simulink model "atrias_boom_nmStand_fullCtrl"  (R2015a)
settings: Solver=ode23t  StartTime=0.0  StopTime=t_end  FixedStep=0.001  MaxStep=1e-3  RelTol=1e-3
InitFcn:
  | addpath('../common/')
  | colors
StartFcn:
  | tic
StopFcn:
  | %stopscript
values from neighbouring files (symbols this model uses):
  A1_notch_f1 = -2*cos(fnotch_f1*sample_time)    [set_control_params.m]
  A2_notch_f1 = 1    [set_control_params.m]
  A_lpf_dtau = 1 + B1_lpf_dtau + B2_lpf_dtau    [set_control_params.m]
  ankle_stiffness = 1/2*pi    (= 1.57079632679)    [mechanical_params.m]
  B1_lpf_dtau = -2*exp(-lpf_damping*fcut_dtau*sample_time)*cos(fcut_dtau*sample_time*sqrt(1-lpf_damping^2))    [set_control_params.m]
  B1_notch_f1 = -2*exp(-notch_damping*fnotch_f1*sample_time)*cos(fnotch_f1*sample_time*sqrt(1-notch_damping^2))    [set_control_params.m]
  B2_lpf_dtau = exp(-2*lpf_damping*fcut_dtau*sample_time)    [set_control_params.m]
  B2_notch_f1 = exp(-2*notch_damping*fnotch_f1*sample_time)    [set_control_params.m]
  b_hmotor = 0    [mechanical_params.m]
  b_leg_spring = 0.075*sqrt(k_leg_spring*0.5*.25^2)    [mechanical_params.m]
  b_rotor = 0*60/(2*pi)*9.725e-5    (= 0)    [mechanical_params.m]
  boom_mount_to_center_diagonal = boom_mount_to_center / cos(pitch_mount_angle)    [mechanical_params.m]    (also in set_control_params.m)
  breakaway_friction = [25 25 25 25]    [mechanical_params.m]
  contactThr = 0.35    [set_control_params.m]
  coulomb_friction = [20 20 20 20]    [mechanical_params.m]
  d_com = (d_hip_com_to_torso_com*m_torso)/(m_torso + num_legs*m_hshaft)    [mechanical_params.m]
  delta_phi_max = 160*pi/180    (= 2.79252680319)    [mechanical_params.m]    (also in set_control_params.m)
  delta_phi_max_buffer = 20*pi/180    (= 0.349065850399)    [set_control_params.m]
  delta_phi_max_dropoff = 2*pi/180    (= 0.0349065850399)    [set_control_params.m]
  delta_phi_min = 25.5*pi/180    (= 0.445058959259)    [mechanical_params.m]    (also in set_control_params.m)
  friction_linear_zone = [0.5 0.5 0.5 0.5].*pi/180    [mechanical_params.m]
  g = 9.803    [mechanical_params.m]    (also in set_control_params.m = 9.81)
  gain_nodes_sea_torque = [0,65,350,700]    [set_control_params.m]
  HIP_MTR_MAX_CONT_TORQUE = HIP_MTR_MAX_CONT_CURRENT*HIP_MOTOR_CONSTANT*HIP_MTR_GEAR_RATIO    (= 86.0016)    [set_control_params.m]
  HIP_MTR_MAX_TORQUE = max_current_hip*Kt_hip*N_h    (= 629.28)    [mechanical_params.m]
  initial_boom_pitch = 0    [mechanical_params.m]
  initial_boom_roll = asin((initial_com_height + boom_mount_to_com + boom_mount_to_center*tan(pitch_mount_angle) - (base_12(2) + yshaft_12(2))) / (l_boom + boom_mount_to_center_diagonal))    [mechanical_params.m]
  initial_boom_yaw = 0    [mechanical_params.m]
  initial_hip_roll = 0*pi/180    (= 0)    [mechanical_params.m]
  initial_winch_angle = -12 * pi/180    (= -0.209439510239)    [mechanical_params.m]
  k_gn = m_total*g/0.01    (= 57041.421916)    [mechanical_params.m]
  k_gt = m_total*g/0.1    (= 5704.1421916)    [mechanical_params.m]
  k_leg_spring = 4118.3    [mechanical_params.m]    (also in set_control_params.m)
  K_notch_f1 = (1+B1_notch_f1+B2_notch_f1)/(1+A1_notch_f1+A2_notch_f1)    [set_control_params.m]
  k_phi = 5000    [mechanical_params.m]
  k_sea = [4118.3 4118.3 4118.3 4118.3]    [set_control_params.m]
  Kb_leg = 0.121    [mechanical_params.m]
  kd_boom_roll_Ctrl = 0    [main_1_nmStand.m]    (also in main_2_nmStand_moveBoom.m)
  kd_lateral = 2*sqrt(kp_lateral*0.8)    [set_control_params.m]
  kd_shin_max = kd_pd_avoid_limits    (= 1000)    [set_control_params.m]
  kd_shin_min = kd_pd_avoid_limits    (= 1000)    [set_control_params.m]
  kd_splay_max = kd_pd_avoid_limits    (= 1000)    [set_control_params.m]
  kd_splay_min = kd_pd_avoid_limits    (= 1000)    [set_control_params.m]
  kd_thigh_max = kd_pd_avoid_limits    (= 1000)    [set_control_params.m]
  kd_thigh_min = kd_pd_avoid_limits    (= 1000)    [set_control_params.m]
  kd_winch = td_winch*kp_winch    (= 989.239577798)    [mechanical_params.m]
  kp_boom_roll_Ctrl = 0    [main_1_nmStand.m]    (also in main_2_nmStand_moveBoom.m)
  kp_lateral = 1000    [set_control_params.m]
  kp_sea_torque = [0.3, 0.3, 6.0, 6.0]    [set_control_params.m]
  kp_shin_max = kp_pd_avoid_limits    (= 5000)    [set_control_params.m]
  kp_shin_min = kp_pd_avoid_limits    (= 5000)    [set_control_params.m]
  kp_splay_max = kp_pd_avoid_limits    (= 5000)    [set_control_params.m]
  kp_splay_min = kp_pd_avoid_limits/10    (= 500)    [set_control_params.m]
  kp_thigh_max = kp_pd_avoid_limits    (= 5000)    [set_control_params.m]
  kp_thigh_min = kp_pd_avoid_limits    (= 5000)    [set_control_params.m]
  kp_winch = winch_gravity_comp/(3*pi/180)    (= 19784.791556)    [mechanical_params.m]
  Kt_leg = 0.121    [mechanical_params.m]
  l_boom = 1.8161    [mechanical_params.m]    (also in set_control_params.m)
  L_leg = 0.102e-3    (= 0.000102)    [mechanical_params.m]
  l_seg = 0.5    [mechanical_params.m]    (also in set_control_params.m)
  l_v = l_seg*cos(min_splay_angle/2)    [set_control_params.m]
  lateral_offset = 0.2    [set_control_params.m]
  lateral_target_angle_right = -6*pi/180    (= -0.10471975512)    [set_control_params.m]
  lateral_transition_force = 150    [set_control_params.m]
  LEG_MTR_MAX_TORQUE = max_current_leg * Kt_leg * N    (= 1210)    [mechanical_params.m]
  loaded_unloaded_torque_threshold = 65*ones(1,4)    [set_control_params.m]
  lowerleg_12 = 0.40    (= 0.4)    [mechanical_params.m]
  m_boom = 4.49    [mechanical_params.m]
  m_fblink = 0.46    [mechanical_params.m]    (also in set_control_params.m)
  m_foot = 0.0857    [mechanical_params.m]
  m_hshaft = 18    [mechanical_params.m]    (also in set_control_params.m = 20)
  m_leg = m_thigh + m_lowerleg + m_shin + m_fblink    (= 2.3438)    [mechanical_params.m]
  m_leg_motor = 18    [set_control_params.m]
  m_lowerleg = 0.4438    [mechanical_params.m]    (also in set_control_params.m)
  m_output_gear = 1e-5    (= 1e-05)    [mechanical_params.m]    (also in set_control_params.m)
  m_rotor = 1e-5    (= 1e-05)    [mechanical_params.m]    (also in set_control_params.m)
  m_shin = 0.75    [mechanical_params.m]    (also in set_control_params.m)
  m_thigh = 0.69    [mechanical_params.m]    (also in set_control_params.m)
  m_torso = 17.5    [mechanical_params.m]    (also in set_control_params.m = 17.9)
  m_total = num_legs*(m_hshaft + m_thigh + m_lowerleg + m_shin + m_fblink + 2*m_gearing) + m_torso    (= 58.18772)    [mechanical_params.m]    (also in set_control_params.m = 62.58772)
  m_virtual_gear = 1e-5    (= 1e-05)    [mechanical_params.m]    (also in set_control_params.m)
  m_yshaft = 12.89    [mechanical_params.m]
  max_current_leg = 200    [mechanical_params.m]
  max_sagittal_loaded_torque = 833    [set_control_params.m]
  max_sagittal_unloaded_torque = 267    [set_control_params.m]
  max_torque_lateral = min(MTR_HIP_MAX_CURRENT, HIP_CURRENT_LIMIT)*HIP_MOTOR_CONSTANT*HIP_MTR_GEAR_RATIO    [set_control_params.m]
  max_voltage_leg = 50    [mechanical_params.m]
  maximum_lateral_angle = 18*pi/180    (= 0.314159265359)    [set_control_params.m]
  min_splay_angle = 45*pi/180    (= 0.785398163397)    [set_control_params.m]
  min_splay_buffer = 1*pi/180    (= 0.0174532925199)    [set_control_params.m]
  min_splay_dropoff = 5*pi/180    (= 0.0872664625997)    [set_control_params.m]
  minimum_lateral_angle = -9.5*pi/180    (= -0.165806278939)    [set_control_params.m]
  mu_hmotor = 0.90    (= 0.9)    [mechanical_params.m]
  mu_motor = 0.85    [mechanical_params.m]
  mu_slide = 0.8    [mechanical_params.m]
  mu_stick = 0.9    [mechanical_params.m]
  N = 50    [mechanical_params.m]
  N_h = r_hip_shaft / r_hip_gearhead    (= 57)    [mechanical_params.m]
  phi_max_collision = -5*pi/180    (= -0.0872664625997)    [mechanical_params.m]
  phi_roll_max = pi + 16*pi/180    (= 3.42084533391)    [mechanical_params.m]
  phi_roll_min = pi - 9*pi/180    (= 2.98451302091)    [mechanical_params.m]
  phi_shin_max = 3*pi/2 + 17.5*pi/180    (= 5.01782159948)    [mechanical_params.m]    (also in set_control_params.m)
  phi_shin_max_buffer = 20*pi/180    (= 0.349065850399)    [set_control_params.m]
  phi_shin_max_dropoff = 2*pi/180    (= 0.0349065850399)    [set_control_params.m]
  phi_shin_min = pi - 45*pi/180    (= 2.35619449019)    [mechanical_params.m]    (also in set_control_params.m)
  phi_shin_min_buffer = 20*pi/180    (= 0.349065850399)    [set_control_params.m]
  phi_shin_min_dropoff = 2*pi/180    (= 0.0349065850399)    [set_control_params.m]
  phi_thigh_max = pi + 45*pi/180    (= 3.92699081699)    [mechanical_params.m]    (also in set_control_params.m)
  phi_thigh_max_buffer = 20*pi/180    (= 0.349065850399)    [set_control_params.m]
  phi_thigh_max_dropoff = 2*pi/180    (= 0.0349065850399)    [set_control_params.m]
  phi_thigh_min = pi/2 - 17.5*pi/180    (= 1.2653637077)    [mechanical_params.m]    (also in set_control_params.m)
  phi_thigh_min_buffer = 20*pi/180    (= 0.349065850399)    [set_control_params.m]
  phi_thigh_min_dropoff = 2*pi/180    (= 0.0349065850399)    [set_control_params.m]
  r_hip_gearhead = 0.009525    [mechanical_params.m]
  r_hip_shaft = 0.542925    [mechanical_params.m]
  R_leg = 0.052    [mechanical_params.m]
  r_rotor = 0.001    [mechanical_params.m]
  r_virtual_gear = N*r_rotor    (= 0.05)    [mechanical_params.m]
  releaseThr = 0.2    [set_control_params.m]
  sample_time = 0.001    [set_control_params.m]
  ... (+19 more)
undefined symbols (not defined in the file or in its folder): A_lpf_velocity, B1_lpf_velocity, B2_lpf_velocity, base_color_d, boom_color_d, c, c_jointstop, CtrlPar_theta0, eref, fblink_color_d, floor_color_d, FmaxBFSH, FmaxGLU, FmaxHAM, FmaxHFL, FmaxRF, FmaxVAS, foot_color_d, FPCtrlPar, hshaft_color_d, j_motor, K, lateral_motor_efficiency, LLCtrlPar, loptBFSH, loptGLU, loptHAM, loptHFL, loptRF, loptVAS, lowerleg_color_d, lslackBFSH, lslackGLU, lslackHAM, lslackHFL, lslackRF, lslackVAS, MidDelay_discrete, Newton, output_sample_time, phi12_max, phi12_min, phi23_max, phi23_min, phimaxRFk, phimaxVAS, phirefBFSH, phirefGLU, phirefHAMh, phirefHAMk, phirefHFL, phirefRFh, phirefRFk, phirefVAS, phiScaleRFk, phiScaleVAS, rad ... (+40)
libraries: sm_lib x210, nesl_utility x140, simulink x58, simulink_extras x26, fl_lib x16, mblibv1 x2, commnoisgen2 x1
(part 18 of 19)

== system atrias_boom_nmStand_fullCtrl/Control/Behavior Control/Virtual Neuromuscular Control/Neural Control Layer/R Swing Phase (sagittal)/kneeii_damp and hold &kneeiii_leg stop &kneeiv_stance preparation ==
  note: Knee Phase i
  CtrlPar : Inport
  a_tgt : Inport  Port=2
  a : Inport  Port=3
  da : Inport  Port=4
  phiH : Inport  Port=5
  phiK : Inport  Port=6
  dphiK : Inport  Port=7
  Enable : EnablePort  StatesWhenEnabling=reset
  Constant1 : Constant  Value=0  OutDataTypeStr=boolean
  Constant2 : Constant  Value=0  OutDataTypeStr=boolean
  Constant3 : Constant  Value=0  OutDataTypeStr=boolean
  Demux1 : Demux  Outputs=2
  Logical Operator : Logic  Operator=NOT  AllPortsSameDT=off  OutDataTypeStr=boolean
  Logical Operator1 : Logic  AllPortsSameDT=off  OutDataTypeStr=boolean
  Mux : Mux  Inputs=3
  Relational Operator : RelationalOperator  Operator=<=  OutDataTypeStr=boolean
  Relational Operator1 : RelationalOperator  Operator=<=  OutDataTypeStr=boolean
  Relational Operator2 : RelationalOperator  OutDataTypeStr=boolean
  S-R Flip-Flop : simulink_extras/Flip Flops/S-R Flip-Flop  initial_condition=0
  S-R Flip-Flop1 : simulink_extras/Flip Flops/S-R Flip-Flop  initial_condition=0
  S-R Flip-Flop2 : simulink_extras/Flip Flops/S-R Flip-Flop  initial_condition=0
  Sum2 : Sum  Inputs=++|  SaturateOnIntegerOverflow=on  InputSameDT=on  OutDataTypeStr=Inherit: Same as first input
  Terminator : Terminator
  Terminator1 : Terminator
  Terminator2 : Terminator
  kneeii_damp and hold : Subsystem  TreatAsAtomicUnit=on
  kneeiii_leg stop : Subsystem  TreatAsAtomicUnit=on
  kneeiv_stance preparation : Subsystem  TreatAsAtomicUnit=on
  parSwKii : Selector  InputPortWidth=Sw_i  Indices=parSwKii_i
  parSwKiii : Selector  InputPortWidth=Sw_i  Indices=parSwKiii_i
  parSwKiv : Selector  InputPortWidth=Sw_i  Indices=parSwKiv_i
  parSwPhii : Selector  InputPortWidth=Sw_i  Indices=parSwPh_i
  phase [M8 M9 M10] : Outport  OutputWhenDisabled=reset  InitialOutput=0
  SRF_Sw_kii : Outport  Port=2  OutputWhenDisabled=reset  InitialOutput=0
  SVAS_Sw_kii : Outport  Port=3  OutputWhenDisabled=reset  InitialOutput=0
  SBFSH_Sw_kii : Outport  Port=4  OutputWhenDisabled=reset  InitialOutput=0
  SHAM_Sw_kiii : Outport  Port=5  OutputWhenDisabled=reset  InitialOutput=0
  SBFSH_Sw_kiii : Outport  Port=6  OutputWhenDisabled=reset  InitialOutput=0
  SHFL_Sw_kiv : Outport  Port=7  OutputWhenDisabled=reset  InitialOutput=0
  SGLU_Sw_kiv : Outport  Port=8  OutputWhenDisabled=reset  InitialOutput=0
  SVAS_Sw_kiv : Outport  Port=9  OutputWhenDisabled=reset  InitialOutput=0
  wires:
  phiK/1 -> kneeiv_stance preparation/4(phiK)
  phiH/1 -> kneeiv_stance preparation/3(phiH)
  dphiK/1 -> kneeii_damp and hold/5(dphiK)
  da/1 -> Relational Operator2/1, kneeii_damp and hold/4(da)
  Sum2/1 -> Relational Operator1/2  "a_thr"
  a/1 -> Relational Operator/1, Relational Operator1/1, kneeiii_leg stop/3(a), kneeii_damp and hold/3("a ")
  Mux/1 -> phase [M8 M9 M10]/1
  Relational Operator2/1 -> Logical Operator1/2
  Logical Operator/1 -> Mux/1, kneeii_damp and hold/Enable
  a_tgt/1 -> kneeiv_stance preparation/2(a_tgt), kneeiii_leg stop/2(a_tgt), kneeii_damp and hold/2(a_tgt), Relational Operator/2, Sum2/1
  kneeiv_stance preparation/3(SVAS_Sw_kiv) -> SVAS_Sw_kiv/1
  kneeiv_stance preparation/2(SGLU_Sw_kiv) -> SGLU_Sw_kiv/1
  kneeiv_stance preparation/1(SHFL_Sw_kiv) -> SHFL_Sw_kiv/1
  kneeiii_leg stop/2(SBFSH_Sw_kiii) -> SBFSH_Sw_kiii/1
  kneeiii_leg stop/1(SHAM_Sw_kiii) -> SHAM_Sw_kiii/1
  kneeii_damp and hold/3(SBFSH_Sw_kii) -> SBFSH_Sw_kii/1
  kneeii_damp and hold/1(SRF_Sw_kii) -> SRF_Sw_kii/1
  parSwKiv/1 -> kneeiv_stance preparation/1(CtrlPar)
  parSwKiii/1 -> kneeiii_leg stop/1(CtrlPar)
  S-R Flip-Flop2/1 -> kneeiv_stance preparation/Enable, Mux/3
  S-R Flip-Flop1/1 -> Logical Operator1/1, kneeiii_leg stop/Enable, Mux/2
  parSwKii/1 -> kneeii_damp and hold/1(CtrlPar)
  S-R Flip-Flop/1 -> Logical Operator/1
  CtrlPar/1 -> parSwKiv/1, parSwKiii/1, parSwKii/1, parSwPhii/1
  Logical Operator1/1 -> S-R Flip-Flop2/1
  S-R Flip-Flop2/2 -> Terminator2/1
  Constant3/1 -> S-R Flip-Flop2/2
  Relational Operator1/1 -> S-R Flip-Flop1/1
  S-R Flip-Flop1/2 -> Terminator1/1
  Constant2/1 -> S-R Flip-Flop1/2
  Relational Operator/1 -> S-R Flip-Flop/1
  S-R Flip-Flop/2 -> Terminator/1
  Constant1/1 -> S-R Flip-Flop/2
  Demux1/1 -> Sum2/2  "Sw_a_del"
  parSwPhii/1 -> Demux1/1
  Demux1/2 -> Relational Operator2/2  "Sw_da_del"
  kneeii_damp and hold/2(SVAS_Sw_kii) -> SVAS_Sw_kii/1

== system atrias_boom_nmStand_fullCtrl/Control/Behavior Control/Virtual Neuromuscular Control/Torque Distribution/mech limit avoidance1/PD Joint Limit ==
  L Mechanical Limit Avoidance Torque : Subsystem
  L scale desired torque : Subsystem
  Mux1 : Mux
  Mux2 : Mux
  R Mechanical Limit Avoidance Torque : Subsystem
  R scale desired torque : Subsystem
  tau_pd_hip_knee [Nm]x4 : Outport
  des_trq_scale x4 : Outport  Port=2
  tag scope: L_scale_hip=global, L_scale_knee=global, Ltau_pd_hip=global, Ltau_pd_knee=global, R_scale_hip=global, R_scale_knee=global, Rtau_pd_hip=global, Rtau_pd_knee=global
  wires:
  L scale desired torque/2(scale_knee) -> [L_scale_knee]
  L scale desired torque/1(scale_hip) -> [L_scale_hip]
  [Lphi_shin] -> L scale desired torque/2(phi_shin [rad])
  [Lphi_thigh] -> L scale desired torque/1(phi_thigh [rad])
  R Mechanical Limit Avoidance Torque/1(tau_pd_hip [Nm]) -> [Rtau_pd_hip]
  L Mechanical Limit Avoidance Torque/2(tau_pd_knee [Nm]) -> [Ltau_pd_knee]
  L Mechanical Limit Avoidance Torque/1(tau_pd_hip [Nm]) -> [Ltau_pd_hip]
  R Mechanical Limit Avoidance Torque/2(tau_pd_knee [Nm]) -> [Rtau_pd_knee]
  Mux2/1 -> tau_pd_hip_knee [Nm]x4/1
  [Rtau_pd_hip] -> Mux2/1
  [Rtau_pd_knee] -> Mux2/2
  [Ltau_pd_hip] -> Mux2/3
  [Ltau_pd_knee] -> Mux2/4
  Mux1/1 -> des_trq_scale x4/1
  [R_scale_hip] -> Mux1/1
  [R_scale_knee] -> Mux1/2
  [L_scale_hip] -> Mux1/3
  [L_scale_knee] -> Mux1/4
  R scale desired torque/2(scale_knee) -> [R_scale_knee]
  R scale desired torque/1(scale_hip) -> [R_scale_hip]
  [Rphi_shin] -> R scale desired torque/2(phi_shin [rad])
  [Rphi_thigh] -> R scale desired torque/1(phi_thigh [rad])
  [Rdphi_shin] -> R Mechanical Limit Avoidance Torque/4(dphi_shin [rad/s])
  [Rdphi_thigh] -> R Mechanical Limit Avoidance Torque/3(dphi_thigh [rad/s])
  [Rphi_shin] -> R Mechanical Limit Avoidance Torque/2(phi_shin [rad])
  [Rphi_thigh] -> R Mechanical Limit Avoidance Torque/1(phi_thigh [rad])
  [Ldphi_shin] -> L Mechanical Limit Avoidance Torque/4(dphi_shin [rad/s])
  [Ldphi_thigh] -> L Mechanical Limit Avoidance Torque/3(dphi_thigh [rad/s])
  [Lphi_shin] -> L Mechanical Limit Avoidance Torque/2(phi_shin [rad])
  [Lphi_thigh] -> L Mechanical Limit Avoidance Torque/1(phi_thigh [rad])

== system atrias_boom_nmStand_fullCtrl/Control/Behavior Control/Virtual Neuromuscular Control/Torque Distribution/mech limit avoidance1/PD Joint Limit1 ==
  Demux : Demux
  Lechanical Limit Avoidance Torques : Subsystem
  Mux1 : Mux
  R Mechanical Limit Avoidance Torque : Subsystem
  R scale desired torque : Subsystem
  R scale desired torque1 : Subsystem
  to hip_knee : MATLAB Function  TreatAsAtomicUnit=on
  tau_pd_hip_knee [Nm]x4 : Outport
  des_trq_scale x4 : Outport  Port=2
  tag scope: L_scale_hip=global, L_scale_knee=global, Ltau_pd_back=global, Ltau_pd_front=global, Ltau_pd_hip=global, Ltau_pd_knee=global, R_scale_hip=global, R_scale_knee=global, Rtau_pd_back=global, Rtau_pd_front=global, Rtau_pd_hip=global, Rtau_pd_knee=global
  wires:
  [Lphi_thigh] -> Lechanical Limit Avoidance Torques/1(phi_thigh [rad])
  [Lphi_shin] -> Lechanical Limit Avoidance Torques/2(phi_shin [rad])
  [Ldphi_thigh] -> Lechanical Limit Avoidance Torques/3(dphi_thigh [rad/s])
  [Ldphi_shin] -> Lechanical Limit Avoidance Torques/4(dphi_shin [rad/s])
  Lechanical Limit Avoidance Torques/1(tau_pd_back [Nm]) -> [Ltau_pd_back]
  Lechanical Limit Avoidance Torques/2(tau_pd_front [Nm]) -> [Ltau_pd_front]
  [Rphi_thigh] -> R Mechanical Limit Avoidance Torque/1(phi_thigh [rad])
  [Rphi_shin] -> R Mechanical Limit Avoidance Torque/2(phi_shin [rad])
  [Rdphi_thigh] -> R Mechanical Limit Avoidance Torque/3(dphi_thigh [rad/s])
  [Rdphi_shin] -> R Mechanical Limit Avoidance Torque/4(dphi_shin [rad/s])
  R Mechanical Limit Avoidance Torque/1(tau_pd_back [Nm]) -> [Rtau_pd_back]
  R Mechanical Limit Avoidance Torque/2(tau_pd_front [Nm]) -> [Rtau_pd_front]
  [Rphi_thigh] -> R scale desired torque/1(phi_thigh [rad])
  [Rphi_shin] -> R scale desired torque/2(phi_shin [rad])
  R scale desired torque/1(scale_hip) -> [R_scale_hip]
  R scale desired torque/2(scale_knee) -> [R_scale_knee]
  [k_R] -> to hip_knee/5(kR)
  [k_L] -> to hip_knee/6(kL)
  [Ltau_pd_front] -> to hip_knee/4(Ltau_front)
  [Ltau_pd_back] -> to hip_knee/3(Ltau_back)
  [Rtau_pd_front] -> to hip_knee/2(Rtau_front)
  [Rtau_pd_back] -> to hip_knee/1(Rtau_back)
  to hip_knee/1(tau_pd_hip_knee) -> tau_pd_hip_knee [Nm]x4/1, Demux/1
  [k_R] -> R scale desired torque/3(k)
  [Lphi_thigh] -> R scale desired torque1/1(phi_thigh [rad])
  [Lphi_shin] -> R scale desired torque1/2(phi_shin [rad])
  R scale desired torque1/1(scale_hip) -> [L_scale_hip]
  R scale desired torque1/2(scale_knee) -> [L_scale_knee]
  [k_L] -> R scale desired torque1/3(k)
  [L_scale_knee] -> Mux1/4
  [L_scale_hip] -> Mux1/3
  [R_scale_knee] -> Mux1/2
  [R_scale_hip] -> Mux1/1
  Mux1/1 -> des_trq_scale x4/1
  Demux/1 -> [Rtau_pd_hip]
  Demux/2 -> [Rtau_pd_knee]
  Demux/3 -> [Ltau_pd_hip]
  Demux/4 -> [Ltau_pd_knee]

== system atrias_boom_nmStand_fullCtrl/Mechanical System Layer/Ground Contact Models/L Back Ground Contact/3D Contact/Kinetic Friction Model/Vector Norm ==
  vec : Inport
  Sqrt : Sqrt  OutputSignalType=real  AlgorithmType=Newton-Raphson  SaturateOnIntegerOverflow=on
  Squares : Math  Operator=square  OutputSignalType=real  SaturateOnIntegerOverflow=on
  Sum of Elements : Sum  Inputs=+
  norm : Outport
  wires:
  vec/1 -> Squares/1
  Sqrt/1 -> norm/1
  Sum of Elements/1 -> Sqrt/1
  Squares/1 -> Sum of Elements/1

== system atrias_boom_nmStand_fullCtrl/Mechanical System Layer/Ground Contact Models/L Back Ground Contact/3D Contact/Static Friction Model/Vector Norm ==
  vec : Inport
  Sqrt : Sqrt  OutputSignalType=real  AlgorithmType=Newton-Raphson  SaturateOnIntegerOverflow=on
  Squares : Math  Operator=square  OutputSignalType=real  SaturateOnIntegerOverflow=on
  Sum of Elements : Sum  Inputs=+
  norm : Outport
  wires:
  vec/1 -> Squares/1
  Sqrt/1 -> norm/1
  Sum of Elements/1 -> Sqrt/1
  Squares/1 -> Sum of Elements/1

== system atrias_boom_nmStand_fullCtrl/Mechanical System Layer/Ground Contact Models/L Front Ground Contact/3D Contact/Kinetic Friction Model/Vector Norm ==
  vec : Inport
  Sqrt : Sqrt  OutputSignalType=real  AlgorithmType=Newton-Raphson  SaturateOnIntegerOverflow=on
  Squares : Math  Operator=square  OutputSignalType=real  SaturateOnIntegerOverflow=on
  Sum of Elements : Sum  Inputs=+
  norm : Outport
  wires:
  vec/1 -> Squares/1
  Sqrt/1 -> norm/1
  Sum of Elements/1 -> Sqrt/1
  Squares/1 -> Sum of Elements/1

== system atrias_boom_nmStand_fullCtrl/Mechanical System Layer/Ground Contact Models/L Front Ground Contact/3D Contact/Static Friction Model/Vector Norm ==
  vec : Inport
  Sqrt : Sqrt  OutputSignalType=real  AlgorithmType=Newton-Raphson  SaturateOnIntegerOverflow=on
  Squares : Math  Operator=square  OutputSignalType=real  SaturateOnIntegerOverflow=on
  Sum of Elements : Sum  Inputs=+
  norm : Outport
  wires:
  vec/1 -> Squares/1
  Sqrt/1 -> norm/1
  Sum of Elements/1 -> Sqrt/1
  Squares/1 -> Sum of Elements/1

== system atrias_boom_nmStand_fullCtrl/Mechanical System Layer/Ground Contact Models/R Back Ground Contact/3D Contact/Kinetic Friction Model/Vector Norm ==
  vec : Inport
  Sqrt : Sqrt  OutputSignalType=real  AlgorithmType=Newton-Raphson  SaturateOnIntegerOverflow=on
  Squares : Math  Operator=square  OutputSignalType=real  SaturateOnIntegerOverflow=on
  Sum of Elements : Sum  Inputs=+
  norm : Outport
  wires:
  vec/1 -> Squares/1
  Sqrt/1 -> norm/1
  Sum of Elements/1 -> Sqrt/1
  Squares/1 -> Sum of Elements/1

== system atrias_boom_nmStand_fullCtrl/Mechanical System Layer/Ground Contact Models/R Back Ground Contact/3D Contact/Static Friction Model/Vector Norm ==
  vec : Inport
  Sqrt : Sqrt  OutputSignalType=real  AlgorithmType=Newton-Raphson  SaturateOnIntegerOverflow=on
  Squares : Math  Operator=square  OutputSignalType=real  SaturateOnIntegerOverflow=on
  Sum of Elements : Sum  Inputs=+
  norm : Outport
  wires:
  vec/1 -> Squares/1
  Sqrt/1 -> norm/1
  Sum of Elements/1 -> Sqrt/1
  Squares/1 -> Sum of Elements/1

== system atrias_boom_nmStand_fullCtrl/Mechanical System Layer/Ground Contact Models/R Front Ground Contact/3D Contact/Kinetic Friction Model/Vector Norm ==
  vec : Inport
  Sqrt : Sqrt  OutputSignalType=real  AlgorithmType=Newton-Raphson  SaturateOnIntegerOverflow=on
  Squares : Math  Operator=square  OutputSignalType=real  SaturateOnIntegerOverflow=on
  Sum of Elements : Sum  Inputs=+
  norm : Outport
  wires:
  vec/1 -> Squares/1
  Sqrt/1 -> norm/1
  Sum of Elements/1 -> Sqrt/1
  Squares/1 -> Sum of Elements/1

== system atrias_boom_nmStand_fullCtrl/Mechanical System Layer/Ground Contact Models/R Front Ground Contact/3D Contact/Static Friction Model/Vector Norm ==
  vec : Inport
  Sqrt : Sqrt  OutputSignalType=real  AlgorithmType=Newton-Raphson  SaturateOnIntegerOverflow=on
  Squares : Math  Operator=square  OutputSignalType=real  SaturateOnIntegerOverflow=on
  Sum of Elements : Sum  Inputs=+
  norm : Outport
  wires:
  vec/1 -> Squares/1
  Sqrt/1 -> norm/1
  Sum of Elements/1 -> Sqrt/1
  Squares/1 -> Sum of Elements/1

== system atrias_boom_nmStand_fullCtrl/Control/Behavior Control/Virtual Neuromuscular Control/Neural Control Layer/L Swing Phase (sagittal)/kneeii_damp and hold &kneeiii_leg stop &kneeiv_stance preparation/kneeii_damp and hold ==
  note: Knee Phase i
  CtrlPar : Inport
  a_tgt : Inport  Port=2
  "a " : Inport  Port=3
  da : Inport  Port=4
  dphiK : Inport  Port=5
  Enable : EnablePort  StatesWhenEnabling=reset
  Demux2 : Demux
  Divide1 : Product
  Divide2 : Product  Inputs=3
  Divide3 : Product
  Divide5 : Product
  Gain3 : Gain  Gain=-1
  Sum2 : Sum  Inputs=|+-  SaturateOnIntegerOverflow=on  InputSameDT=on  OutDataTypeStr=Inherit: Same as first input
  Sum4 : Sum  Inputs=+-|  SaturateOnIntegerOverflow=on  InputSameDT=on  OutDataTypeStr=Inherit: Same as first input
  Sum7 : Sum  Inputs=++|  SaturateOnIntegerOverflow=on  InputSameDT=on  OutDataTypeStr=Inherit: Same as first input
  negative half : Saturate  UpperLimit=0  LowerLimit=-inf  ZeroCross=off
  positive half{,1..3} (4 alike) : Saturate  UpperLimit=inf  LowerLimit=0  ZeroCross=off
  SRF_Sw_kii : Outport  OutputWhenDisabled=reset  InitialOutput=0
  SVAS_Sw_kii : Outport  Port=2  OutputWhenDisabled=reset  InitialOutput=0
  SBFSH_Sw_kii : Outport  Port=3  OutputWhenDisabled=reset  InitialOutput=0
  wires:
  Demux2/4 -> Divide1/2  "Sw_dphiKGain_BFSH"
  Demux2/1 -> Divide5/2  "Sw_dphiKGain_RF"
  da/1 -> Sum7/2
  dphiK/1 -> negative half/1, Sum7/1, positive half/1
  a_tgt/1 -> Sum2/1
  Divide2/1 -> SBFSH_Sw_kii/1
  Sum2/1 -> positive half2/1
  "a "/1 -> Sum2/2
  positive half2/1 -> Divide2/3
  Sum7/1 -> positive half1/1
  positive half1/1 -> Divide2/2
  Divide1/1 -> Divide2/1
  positive half/1 -> Divide1/1
  Divide5/1 -> SRF_Sw_kii/1, Sum4/1
  CtrlPar/1 -> Demux2/1
  negative half/1 -> Gain3/1
  Gain3/1 -> Divide5/1
  positive half3/1 -> Divide3/1
  Sum4/1 -> positive half3/1
  Demux2/2 -> Sum4/2  "Sw_SRF_thr"
  Demux2/3 -> Divide3/2  "Sw_SGainRF_VAS"
  Divide3/1 -> SVAS_Sw_kii/1

== system atrias_boom_nmStand_fullCtrl/Control/Behavior Control/Virtual Neuromuscular Control/Neural Control Layer/L Swing Phase (sagittal)/kneeii_damp and hold &kneeiii_leg stop &kneeiv_stance preparation/kneeiii_leg stop ==
  note: Knee Phase iii
  CtrlPar : Inport
  a_tgt : Inport  Port=2
  a : Inport  Port=3
  Enable : EnablePort  StatesWhenEnabling=reset
  Demux2 : Demux
  Divide1 : Product
  Divide5 : Product
  Sum1 : Sum  Inputs=+-|  SaturateOnIntegerOverflow=on  InputSameDT=on  OutDataTypeStr=Inherit: Same as first input
  Sum2 : Sum  Inputs=++|  SaturateOnIntegerOverflow=on  InputSameDT=on  OutDataTypeStr=Inherit: Same as first input
  Sum4 : Sum  Inputs=+-|  SaturateOnIntegerOverflow=on  InputSameDT=on  OutDataTypeStr=Inherit: Same as first input
  positive half1 : Saturate  UpperLimit=inf  LowerLimit=0  ZeroCross=off
  positive half2 : Saturate  UpperLimit=inf  LowerLimit=0  ZeroCross=off
  SHAM_Sw_kiii : Outport  OutputWhenDisabled=reset  InitialOutput=0
  SBFSH_Sw_kiii : Outport  Port=2  OutputWhenDisabled=reset  InitialOutput=0
  wires:
  Demux2/1 -> Sum2/2  "Sw_a_del"
  a/1 -> Sum1/2
  Divide1/1 -> SBFSH_Sw_kiii/1
  Demux2/4 -> Divide1/2  "Sw_SGainHAM_BFSH"
  positive half1/1 -> Divide1/1
  Demux2/3 -> Sum4/2  "SHAM_thr"
  Sum4/1 -> positive half1/1
  Divide5/1 -> SHAM_Sw_kiii/1, Sum4/1  "S_HAM"
  Demux2/2 -> Divide5/2  "Sw_alpGain_HAM"
  Sum2/1 -> Sum1/1  "a_thr"
  a_tgt/1 -> Sum2/1
  positive half2/1 -> Divide5/1  "del_alp"
  Sum1/1 -> positive half2/1  "del_alp"
  CtrlPar/1 -> Demux2/1

== system atrias_boom_nmStand_fullCtrl/Control/Behavior Control/Virtual Neuromuscular Control/Neural Control Layer/L Swing Phase (sagittal)/kneeii_damp and hold &kneeiii_leg stop &kneeiv_stance preparation/kneeiv_stance preparation ==
  note: Knee Phase iii
  CtrlPar : Inport
  a_tgt : Inport  Port=2
  phiH : Inport  Port=3
  phiK : Inport  Port=4
  Enable : EnablePort  StatesWhenEnabling=reset
  Constant5 : Constant  Value=pi/2
  Demux1 : Demux
  Divide3 : Product
  Divide5 : Product
  Divide6 : Product
  Sum1 : Sum  Inputs=-+|  SaturateOnIntegerOverflow=on  InputSameDT=on  OutDataTypeStr=Inherit: Same as first input
  Sum2 : Sum  Inputs=++|  SaturateOnIntegerOverflow=on  InputSameDT=on  OutDataTypeStr=Inherit: Same as first input
  Sum9 : Sum  Inputs=+-|  SaturateOnIntegerOverflow=on  InputSameDT=on  OutDataTypeStr=Inherit: Same as first input
  positive half2 : Saturate  UpperLimit=inf  LowerLimit=0  ZeroCross=off
  positive half3 : Saturate  UpperLimit=inf  LowerLimit=0  ZeroCross=off
  SHFL_Sw_kiv : Outport  OutputWhenDisabled=reset  InitialOutput=0
  SGLU_Sw_kiv : Outport  Port=2  OutputWhenDisabled=reset  InitialOutput=0
  SVAS_Sw_kiv : Outport  Port=3  OutputWhenDisabled=reset  InitialOutput=0
  wires:
  Demux1/4 -> Divide6/2
  Demux1/3 -> Sum9/1
  Demux1/2 -> Divide3/1
  Demux1/1 -> Divide5/2
  phiH/1 -> Sum1/2
  Divide6/1 -> SVAS_Sw_kiv/1
  positive half3/1 -> Divide6/1
  phiK/1 -> Sum9/2
  Sum9/1 -> positive half3/1
  Divide3/1 -> SGLU_Sw_kiv/1
  positive half2/1 -> Divide5/1, Divide3/2
  Divide5/1 -> SHFL_Sw_kiv/1
  Sum2/1 -> Sum1/1
  Constant5/1 -> Sum2/1
  a_tgt/1 -> Sum2/2
  Sum1/1 -> positive half2/1
  CtrlPar/1 -> Demux1/1

== system atrias_boom_nmStand_fullCtrl/Control/Behavior Control/Virtual Neuromuscular Control/Neural Control Layer/R Swing Phase (sagittal)/kneeii_damp and hold &kneeiii_leg stop &kneeiv_stance preparation/kneeii_damp and hold ==
  note: Knee Phase i
  CtrlPar : Inport
  a_tgt : Inport  Port=2
  "a " : Inport  Port=3
  da : Inport  Port=4
  dphiK : Inport  Port=5
  Enable : EnablePort  StatesWhenEnabling=reset
  Demux2 : Demux
  Divide1 : Product
  Divide2 : Product  Inputs=3
  Divide3 : Product
  Divide5 : Product
  Gain3 : Gain  Gain=-1
  Sum2 : Sum  Inputs=|+-  SaturateOnIntegerOverflow=on  InputSameDT=on  OutDataTypeStr=Inherit: Same as first input
  Sum4 : Sum  Inputs=+-|  SaturateOnIntegerOverflow=on  InputSameDT=on  OutDataTypeStr=Inherit: Same as first input
  Sum7 : Sum  Inputs=++|  SaturateOnIntegerOverflow=on  InputSameDT=on  OutDataTypeStr=Inherit: Same as first input
  negative half : Saturate  UpperLimit=0  LowerLimit=-inf  ZeroCross=off
  positive half{,1..3} (4 alike) : Saturate  UpperLimit=inf  LowerLimit=0  ZeroCross=off
  SRF_Sw_kii : Outport  OutputWhenDisabled=reset  InitialOutput=0
  SVAS_Sw_kii : Outport  Port=2  OutputWhenDisabled=reset  InitialOutput=0
  SBFSH_Sw_kii : Outport  Port=3  OutputWhenDisabled=reset  InitialOutput=0
  wires:
  Demux2/4 -> Divide1/2  "Sw_dphiKGain_BFSH"
  Demux2/1 -> Divide5/2  "Sw_dphiKGain_RF"
  da/1 -> Sum7/2
  dphiK/1 -> negative half/1, Sum7/1, positive half/1
  a_tgt/1 -> Sum2/1
  Divide2/1 -> SBFSH_Sw_kii/1
  Sum2/1 -> positive half2/1
  "a "/1 -> Sum2/2
  positive half2/1 -> Divide2/3
  Sum7/1 -> positive half1/1
  positive half1/1 -> Divide2/2
  Divide1/1 -> Divide2/1
  positive half/1 -> Divide1/1
  Divide5/1 -> SRF_Sw_kii/1, Sum4/1
  CtrlPar/1 -> Demux2/1
  negative half/1 -> Gain3/1
  Gain3/1 -> Divide5/1
  positive half3/1 -> Divide3/1
  Sum4/1 -> positive half3/1
  Demux2/2 -> Sum4/2  "Sw_SRF_thr"
  Demux2/3 -> Divide3/2  "Sw_SGainRF_VAS"
  Divide3/1 -> SVAS_Sw_kii/1

== system atrias_boom_nmStand_fullCtrl/Control/Behavior Control/Virtual Neuromuscular Control/Neural Control Layer/R Swing Phase (sagittal)/kneeii_damp and hold &kneeiii_leg stop &kneeiv_stance preparation/kneeiii_leg stop ==
  note: Knee Phase iii
  CtrlPar : Inport
  a_tgt : Inport  Port=2
  a : Inport  Port=3
  Enable : EnablePort  StatesWhenEnabling=reset
  Demux2 : Demux
  Divide1 : Product
  Divide5 : Product
  Sum1 : Sum  Inputs=+-|  SaturateOnIntegerOverflow=on  InputSameDT=on  OutDataTypeStr=Inherit: Same as first input
  Sum2 : Sum  Inputs=++|  SaturateOnIntegerOverflow=on  InputSameDT=on  OutDataTypeStr=Inherit: Same as first input
  Sum4 : Sum  Inputs=+-|  SaturateOnIntegerOverflow=on  InputSameDT=on  OutDataTypeStr=Inherit: Same as first input
  positive half1 : Saturate  UpperLimit=inf  LowerLimit=0  ZeroCross=off
  positive half2 : Saturate  UpperLimit=inf  LowerLimit=0  ZeroCross=off
  SHAM_Sw_kiii : Outport  OutputWhenDisabled=reset  InitialOutput=0
  SBFSH_Sw_kiii : Outport  Port=2  OutputWhenDisabled=reset  InitialOutput=0
  wires:
  Demux2/1 -> Sum2/2  "Sw_a_del"
  a/1 -> Sum1/2
  Divide1/1 -> SBFSH_Sw_kiii/1
  Demux2/4 -> Divide1/2  "Sw_SGainHAM_BFSH"
  positive half1/1 -> Divide1/1
  Demux2/3 -> Sum4/2  "SHAM_thr"
  Sum4/1 -> positive half1/1
  Divide5/1 -> SHAM_Sw_kiii/1, Sum4/1  "S_HAM"
  Demux2/2 -> Divide5/2  "Sw_alpGain_HAM"
  Sum2/1 -> Sum1/1  "a_thr"
  a_tgt/1 -> Sum2/1
  positive half2/1 -> Divide5/1  "del_alp"
  Sum1/1 -> positive half2/1  "del_alp"
  CtrlPar/1 -> Demux2/1

== system atrias_boom_nmStand_fullCtrl/Control/Behavior Control/Virtual Neuromuscular Control/Neural Control Layer/R Swing Phase (sagittal)/kneeii_damp and hold &kneeiii_leg stop &kneeiv_stance preparation/kneeiv_stance preparation ==
  note: Knee Phase iii
  CtrlPar : Inport
  a_tgt : Inport  Port=2
  phiH : Inport  Port=3
  phiK : Inport  Port=4
  Enable : EnablePort  StatesWhenEnabling=reset
  Constant5 : Constant  Value=pi/2
  Demux1 : Demux
  Divide3 : Product
  Divide5 : Product
  Divide6 : Product
  Sum1 : Sum  Inputs=-+|  SaturateOnIntegerOverflow=on  InputSameDT=on  OutDataTypeStr=Inherit: Same as first input
  Sum2 : Sum  Inputs=++|  SaturateOnIntegerOverflow=on  InputSameDT=on  OutDataTypeStr=Inherit: Same as first input
  Sum9 : Sum  Inputs=+-|  SaturateOnIntegerOverflow=on  InputSameDT=on  OutDataTypeStr=Inherit: Same as first input
  positive half2 : Saturate  UpperLimit=inf  LowerLimit=0  ZeroCross=off
  positive half3 : Saturate  UpperLimit=inf  LowerLimit=0  ZeroCross=off
  SHFL_Sw_kiv : Outport  OutputWhenDisabled=reset  InitialOutput=0
  SGLU_Sw_kiv : Outport  Port=2  OutputWhenDisabled=reset  InitialOutput=0
  SVAS_Sw_kiv : Outport  Port=3  OutputWhenDisabled=reset  InitialOutput=0
  wires:
  Demux1/4 -> Divide6/2
  Demux1/3 -> Sum9/1
  Demux1/2 -> Divide3/1
  Demux1/1 -> Divide5/2
  phiH/1 -> Sum1/2
  Divide6/1 -> SVAS_Sw_kiv/1
  positive half3/1 -> Divide6/1
  phiK/1 -> Sum9/2
  Sum9/1 -> positive half3/1
  Divide3/1 -> SGLU_Sw_kiv/1
  positive half2/1 -> Divide5/1, Divide3/2
  Divide5/1 -> SHFL_Sw_kiv/1
  Sum2/1 -> Sum1/1
  Constant5/1 -> Sum2/1
  a_tgt/1 -> Sum2/2
  Sum1/1 -> positive half2/1
  CtrlPar/1 -> Demux1/1

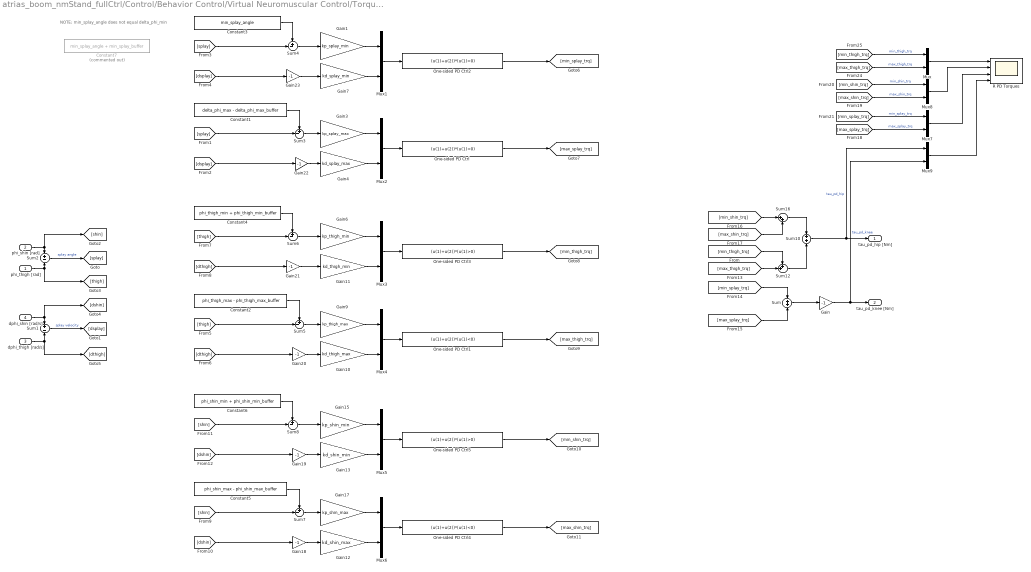
== system atrias_boom_nmStand_fullCtrl/Control/Behavior Control/Virtual Neuromuscular Control/Torque Distribution/mech limit avoidance1/PD Joint Limit/L Mechanical Limit Avoidance Torque ==
  note: NOTE: min_splay_angle does not equal delta_phi_min
  phi_thigh [rad] : Inport
  phi_shin [rad] : Inport  Port=2
  dphi_thigh [rad/s] : Inport  Port=3
  dphi_shin [rad/s] : Inport  Port=4
  Constant1 : Constant  Value=delta_phi_max - delta_phi_max_buffer
  Constant2 : Constant  Value=phi_thigh_max - phi_thigh_max_buffer
  Constant3 : Constant  Value=min_splay_angle
  Constant4 : Constant  Value=phi_thigh_min + phi_thigh_min_buffer
  Constant5 : Constant  Value=phi_shin_max - phi_shin_max_buffer
  Constant6 : Constant  Value=phi_shin_min + phi_shin_min_buffer
  Constant7 : Constant  Commented=on  Value=min_splay_angle + min_splay_buffer
  Gain{,18..23} (7 alike) : Gain  Gain=-1
  Gain1 : Gain  Gain=kp_splay_min
  Gain10 : Gain  Gain=kd_thigh_max
  Gain11 : Gain  Gain=kd_thigh_min
  Gain12 : Gain  Gain=kd_shin_max
  Gain13 : Gain  Gain=kd_shin_min
  Gain15 : Gain  Gain=kp_shin_min
  Gain17 : Gain  Gain=kp_shin_max
  Gain3 : Gain  Gain=kp_splay_max
  Gain4 : Gain  Gain=kd_splay_max
  Gain6 : Gain  Gain=kp_thigh_min
  Gain7 : Gain  Gain=kd_splay_min
  Gain9 : Gain  Gain=kp_thigh_max
  Mux{,1..9} (10 alike) : Mux  Inputs=2
  One-sided PD Ctrl : Fcn  Expr=(u(1)+u(2))*(u(1)<0)
  One-sided PD Ctrl1 : Fcn  Expr=(u(1)+u(2))*(u(1)<0)
  One-sided PD Ctrl2 : Fcn  Expr=(u(1)+u(2))*(u(1)>0)
  One-sided PD Ctrl3 : Fcn  Expr=(u(1)+u(2))*(u(1)>0)
  One-sided PD Ctrl4 : Fcn  Expr=(u(1)+u(2))*(u(1)<0)
  One-sided PD Ctrl5 : Fcn  Expr=(u(1)+u(2))*(u(1)>0)
  R PD Torques : Scope  NumInputPorts=4
      settings: ShowLegends=on  TimeRange=2.5  YMin=-100~-5e+07~-1e+07~-5  YMax=100~1e+07~5e+07~5  SaveName=ScopeData5
  Sum : Sum
  Sum1 : Sum  Inputs=+-
  Sum10 : Sum
  Sum12 : Sum  Inputs=++|
  Sum16 : Sum  Inputs=|++
  Sum2 : Sum  Inputs=+-
  Sum{3..8} (6 alike) : Sum  Inputs=+-|
  tau_pd_hip [Nm] : Outport
  tau_pd_knee [Nm] : Outport  Port=2
  wires:
  One-sided PD Ctrl4/1 -> [max_shin_trq]
  One-sided PD Ctrl5/1 -> [min_shin_trq]
  One-sided PD Ctrl1/1 -> [max_thigh_trq]
  One-sided PD Ctrl3/1 -> [min_thigh_trq]
  One-sided PD Ctrl/1 -> [max_splay_trq]
  Gain23/1 -> Gain7/1
  Gain22/1 -> Gain4/1
  Gain21/1 -> Gain11/1
  Gain20/1 -> Gain10/1
  Gain19/1 -> Gain13/1
  Gain18/1 -> Gain12/1
  [max_splay_trq] -> Mux7/2  "max_splay_trq"
  [min_splay_trq] -> Mux7/1  "min_splay_trq"
  Mux7/1 -> R PD Torques/3
  Mux8/1 -> R PD Torques/2
  [max_shin_trq] -> Mux8/2  "max_shin_trq"
  [min_shin_trq] -> Mux8/1  "min_shin_trq"
  Mux/1 -> R PD Torques/1
  [max_thigh_trq] -> Mux/2  "max_thigh_trq"
  [min_thigh_trq] -> Mux/1  "min_thigh_trq"
  One-sided PD Ctrl2/1 -> [min_splay_trq]
  Mux6/1 -> One-sided PD Ctrl4/1
  Constant5/1 -> Sum7/1
  Sum7/1 -> Gain17/1
  Gain17/1 -> Mux6/1
  Gain12/1 -> Mux6/2
  [shin] -> Sum7/2
  [dshin] -> Gain18/1
  Mux5/1 -> One-sided PD Ctrl5/1
  Constant6/1 -> Sum8/1
  Sum8/1 -> Gain15/1
  Gain15/1 -> Mux5/1
  Gain13/1 -> Mux5/2
  [shin] -> Sum8/2
  [dshin] -> Gain19/1
  Mux4/1 -> One-sided PD Ctrl1/1
  Constant2/1 -> Sum5/1
  Sum5/1 -> Gain9/1
  Gain9/1 -> Mux4/1
  Gain10/1 -> Mux4/2
  [thigh] -> Sum5/2
  [dthigh] -> Gain20/1
  Mux3/1 -> One-sided PD Ctrl3/1
  Constant4/1 -> Sum6/1
  Sum6/1 -> Gain6/1
  Gain6/1 -> Mux3/1
  Gain11/1 -> Mux3/2
  [thigh] -> Sum6/2
  [dthigh] -> Gain21/1
  Mux2/1 -> One-sided PD Ctrl/1
  Constant1/1 -> Sum3/1
  Sum3/1 -> Gain3/1
  Gain3/1 -> Mux2/1
  Gain4/1 -> Mux2/2
  [splay] -> Sum3/2
  [dsplay] -> Gain22/1
  Mux1/1 -> One-sided PD Ctrl2/1
  Constant3/1 -> Sum4/1
  Sum4/1 -> Gain1/1
  Gain1/1 -> Mux1/1
  Gain7/1 -> Mux1/2
  [splay] -> Sum4/2
  [dsplay] -> Gain23/1
  Sum1/1 -> [dsplay]  "splay velocity"
  Sum2/1 -> [splay]  "splay angle"
  phi_thigh [rad]/1 -> Sum2/2, [thigh]
  phi_shin [rad]/1 -> Sum2/1, [shin]
  dphi_thigh [rad/s]/1 -> Sum1/2, [dthigh]
  dphi_shin [rad/s]/1 -> Sum1/1, [dshin]
  [min_splay_trq] -> Sum/1
  [max_splay_trq] -> Sum/2
  Sum/1 -> Gain/1
  Gain/1 -> Mux9/2, tau_pd_knee [Nm]/1  "tau_pd_knee"
  [max_thigh_trq] -> Sum12/2
  [min_thigh_trq] -> Sum12/1
  [min_shin_trq] -> Sum16/1
  [max_shin_trq] -> Sum16/2
  Sum16/1 -> Sum10/1
  Sum12/1 -> Sum10/2
  Sum10/1 -> Mux9/1, tau_pd_hip [Nm]/1  "tau_pd_hip"
  Mux9/1 -> R PD Torques/4

== system atrias_boom_nmStand_fullCtrl/Control/Behavior Control/Virtual Neuromuscular Control/Torque Distribution/mech limit avoidance1/PD Joint Limit/L scale desired torque ==
  note: NOTE: min_splay_angle does not equal delta_phi_min
  phi_thigh [rad] : Inport
  phi_shin [rad] : Inport  Port=2
  Constant : Constant
  Constant1 : Constant  Value=delta_phi_max - delta_phi_max_buffer
  Constant10 : Constant  Value=phi_thigh_max_buffer
  Constant11 : Constant  Value=phi_shin_min_buffer
  Constant12 : Constant  Value=phi_shin_max_buffer
  Constant13 : Constant
  Constant2 : Constant  Value=phi_thigh_max - phi_thigh_max_buffer
  Constant3 : Constant  Value=min_splay_angle
  Constant4 : Constant  Value=phi_thigh_min + phi_thigh_min_buffer
  Constant5 : Constant  Value=phi_shin_max - phi_shin_max_buffer
  Constant6 : Constant  Value=phi_shin_min + phi_shin_min_buffer
  Constant7 : Constant  Value=min_splay_angle - delta_phi_min
  Constant8 : Constant  Value=delta_phi_max_buffer
  Constant9 : Constant  Value=phi_thigh_min_buffer
  Divide{,1..5} (6 alike) : Product  Inputs=/*
  Gain : Gain  Gain=-1
  Gain1 : Gain  Gain=-1
  Gain2 : Gain  Gain=-1
  L scale hip/knee : Scope  NumInputPorts=4
      settings: ShowLegends=on  TimeRange=2.5  YMin=-100~-5e+07~-1e+07~-5  YMax=100~1e+07~5e+07~5  SaveName=ScopeData5
  Mux{,3,7..8} (4 alike) : Mux  Inputs=2
  Sum : Sum  Inputs=|+-
  Sum1 : Sum  Inputs=-+|
  Sum2 : Sum  Inputs=+-
  Sum{3..8} (6 alike) : Sum  Inputs=+-|
  [0,1]{,1..5} (6 alike) : Saturate  UpperLimit=1  LowerLimit=0
  max : MinMax  Function=max  Inputs=2
  max1 : MinMax  Function=max  Inputs=4
  scale_hip : Outport
  scale_knee : Outport  Port=2
  wires:
  max/1 -> Sum1/1
  max1/1 -> Sum/2
  phi_shin [rad]/1 -> [shin], Sum2/1
  phi_thigh [rad]/1 -> [thigh], Sum2/2
  Sum2/1 -> [splay]  "splay angle"
  [splay] -> Sum4/2
  Constant3/1 -> Sum4/1
  [splay] -> Sum3/2
  Constant1/1 -> Sum3/1
  [thigh] -> Sum6/2
  Constant4/1 -> Sum6/1
  [thigh] -> Sum5/2
  Constant2/1 -> Sum5/1
  [shin] -> Sum8/2
  Constant6/1 -> Sum8/1
  [shin] -> Sum7/2
  Constant5/1 -> Sum7/1
  [min_thigh_scale] -> Mux/1  "min_thigh_scale"
  [max_thigh_scale] -> Mux/2  "max_thigh_scale"
  Mux/1 -> L scale hip/knee/1
  [min_shin_scale] -> Mux8/1  "min_shin_scale"
  [max_shin_scale] -> Mux8/2  "max_shin_scale"
  Mux8/1 -> L scale hip/knee/2
  Mux7/1 -> L scale hip/knee/3
  [min_splay_scale] -> Mux7/1  "min_splay_scale"
  [max_splay_scale] -> Mux7/2  "max_splay_scale"
  Sum/1 -> Mux3/1, scale_hip/1
  Constant/1 -> Sum/1
  Constant7/1 -> Divide/1
  Sum4/1 -> Divide/2
  Divide/1 -> "[0,1]"/1
  "[0,1]"/1 -> [min_splay_scale]
  Divide1/1 -> "[0,1]1"/1
  "[0,1]1"/1 -> [max_splay_scale]
  Sum3/1 -> Gain/1
  Constant8/1 -> Divide1/1
  Gain/1 -> Divide1/2
  Divide2/1 -> "[0,1]2"/1
  "[0,1]2"/1 -> [min_thigh_scale]
  Sum6/1 -> Divide2/2
  Constant9/1 -> Divide2/1
  Divide3/1 -> "[0,1]3"/1
  "[0,1]3"/1 -> [max_thigh_scale]
  Gain1/1 -> Divide3/2
  Sum5/1 -> Gain1/1
  Constant10/1 -> Divide3/1
  Divide4/1 -> "[0,1]4"/1
  "[0,1]4"/1 -> [min_shin_scale]
  Sum8/1 -> Divide4/2
  Constant11/1 -> Divide4/1
  Divide5/1 -> "[0,1]5"/1
  "[0,1]5"/1 -> [max_shin_scale]
  Sum7/1 -> Gain2/1
  Constant12/1 -> Divide5/1
  Gain2/1 -> Divide5/2
  Constant13/1 -> Sum1/2
  Sum1/1 -> Mux3/2, scale_knee/1
  Mux3/1 -> L scale hip/knee/4
  [min_splay_scale] -> max/1
  [max_splay_scale] -> max/2
  [max_thigh_scale] -> max1/4
  [min_thigh_scale] -> max1/3
  [max_shin_scale] -> max1/2
  [min_shin_scale] -> max1/1

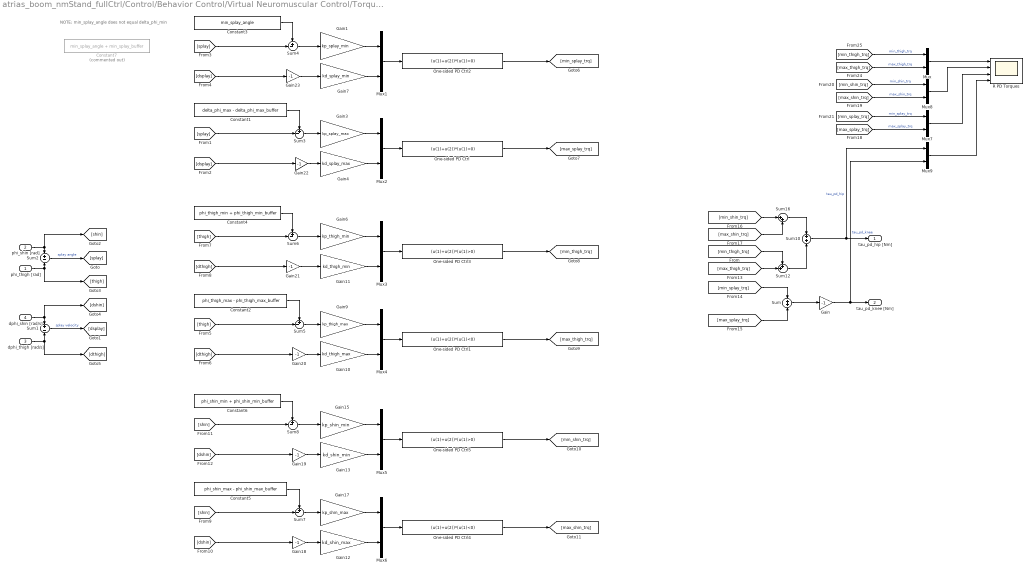
== system atrias_boom_nmStand_fullCtrl/Control/Behavior Control/Virtual Neuromuscular Control/Torque Distribution/mech limit avoidance1/PD Joint Limit/R Mechanical Limit Avoidance Torque ==
  note: NOTE: min_splay_angle does not equal delta_phi_min
  phi_thigh [rad] : Inport
  phi_shin [rad] : Inport  Port=2
  dphi_thigh [rad/s] : Inport  Port=3
  dphi_shin [rad/s] : Inport  Port=4
  Constant1 : Constant  Value=delta_phi_max - delta_phi_max_buffer
  Constant2 : Constant  Value=phi_thigh_max - phi_thigh_max_buffer
  Constant3 : Constant  Value=min_splay_angle
  Constant4 : Constant  Value=phi_thigh_min + phi_thigh_min_buffer
  Constant5 : Constant  Value=phi_shin_max - phi_shin_max_buffer
  Constant6 : Constant  Value=phi_shin_min + phi_shin_min_buffer
  Constant7 : Constant  Commented=on  Value=min_splay_angle + min_splay_buffer
  Gain{,18..23} (7 alike) : Gain  Gain=-1
  Gain1 : Gain  Gain=kp_splay_min
  Gain10 : Gain  Gain=kd_thigh_max
  Gain11 : Gain  Gain=kd_thigh_min
  Gain12 : Gain  Gain=kd_shin_max
  Gain13 : Gain  Gain=kd_shin_min
  Gain15 : Gain  Gain=kp_shin_min
  Gain17 : Gain  Gain=kp_shin_max
  Gain3 : Gain  Gain=kp_splay_max
  Gain4 : Gain  Gain=kd_splay_max
  Gain6 : Gain  Gain=kp_thigh_min
  Gain7 : Gain  Gain=kd_splay_min
  Gain9 : Gain  Gain=kp_thigh_max
  Mux{,1..9} (10 alike) : Mux  Inputs=2
  One-sided PD Ctrl : Fcn  Expr=(u(1)+u(2))*(u(1)<0)
  One-sided PD Ctrl1 : Fcn  Expr=(u(1)+u(2))*(u(1)<0)
  One-sided PD Ctrl2 : Fcn  Expr=(u(1)+u(2))*(u(1)>0)
  One-sided PD Ctrl3 : Fcn  Expr=(u(1)+u(2))*(u(1)>0)
  One-sided PD Ctrl4 : Fcn  Expr=(u(1)+u(2))*(u(1)<0)
  One-sided PD Ctrl5 : Fcn  Expr=(u(1)+u(2))*(u(1)>0)
  R PD Torques : Scope  NumInputPorts=4
      settings: ShowLegends=on  TimeRange=2.5  YMin=-100~-5e+07~-1e+07~-5  YMax=100~1e+07~5e+07~5  SaveName=ScopeData5
  Sum : Sum
  Sum1 : Sum  Inputs=+-
  Sum10 : Sum
  Sum12 : Sum  Inputs=++|
  Sum16 : Sum  Inputs=|++
  Sum2 : Sum  Inputs=+-
  Sum{3..8} (6 alike) : Sum  Inputs=+-|
  tau_pd_hip [Nm] : Outport
  tau_pd_knee [Nm] : Outport  Port=2
  wires:
  Mux9/1 -> R PD Torques/4
  Sum10/1 -> tau_pd_hip [Nm]/1, Mux9/1  "tau_pd_hip"
  Sum12/1 -> Sum10/2
  Sum16/1 -> Sum10/1
  [max_shin_trq] -> Sum16/2
  [min_shin_trq] -> Sum16/1
  [min_thigh_trq] -> Sum12/1
  [max_thigh_trq] -> Sum12/2
  Gain/1 -> tau_pd_knee [Nm]/1, Mux9/2  "tau_pd_knee"
  Sum/1 -> Gain/1
  [max_splay_trq] -> Sum/2
  [min_splay_trq] -> Sum/1
  dphi_shin [rad/s]/1 -> [dshin], Sum1/1
  dphi_thigh [rad/s]/1 -> [dthigh], Sum1/2
  phi_shin [rad]/1 -> [shin], Sum2/1
  phi_thigh [rad]/1 -> [thigh], Sum2/2
  Sum2/1 -> [splay]  "splay angle"
  Sum1/1 -> [dsplay]  "splay velocity"
  [dsplay] -> Gain23/1
  [splay] -> Sum4/2
  Gain7/1 -> Mux1/2
  Gain1/1 -> Mux1/1
  Sum4/1 -> Gain1/1
  Constant3/1 -> Sum4/1
  Mux1/1 -> One-sided PD Ctrl2/1
  [dsplay] -> Gain22/1
  [splay] -> Sum3/2
  Gain4/1 -> Mux2/2
  Gain3/1 -> Mux2/1
  Sum3/1 -> Gain3/1
  Constant1/1 -> Sum3/1
  Mux2/1 -> One-sided PD Ctrl/1
  [dthigh] -> Gain21/1
  [thigh] -> Sum6/2
  Gain11/1 -> Mux3/2
  Gain6/1 -> Mux3/1
  Sum6/1 -> Gain6/1
  Constant4/1 -> Sum6/1
  Mux3/1 -> One-sided PD Ctrl3/1
  [dthigh] -> Gain20/1
  [thigh] -> Sum5/2
  Gain10/1 -> Mux4/2
  Gain9/1 -> Mux4/1
  Sum5/1 -> Gain9/1
  Constant2/1 -> Sum5/1
  Mux4/1 -> One-sided PD Ctrl1/1
  [dshin] -> Gain19/1
  [shin] -> Sum8/2
  Gain13/1 -> Mux5/2
  Gain15/1 -> Mux5/1
  Sum8/1 -> Gain15/1
  Constant6/1 -> Sum8/1
  Mux5/1 -> One-sided PD Ctrl5/1
  [dshin] -> Gain18/1
  [shin] -> Sum7/2
  Gain12/1 -> Mux6/2
  Gain17/1 -> Mux6/1
  Sum7/1 -> Gain17/1
  Constant5/1 -> Sum7/1
  Mux6/1 -> One-sided PD Ctrl4/1
  One-sided PD Ctrl2/1 -> [min_splay_trq]
  [min_thigh_trq] -> Mux/1  "min_thigh_trq"
  [max_thigh_trq] -> Mux/2  "max_thigh_trq"
  Mux/1 -> R PD Torques/1
  [min_shin_trq] -> Mux8/1  "min_shin_trq"
  [max_shin_trq] -> Mux8/2  "max_shin_trq"
  Mux8/1 -> R PD Torques/2
  Mux7/1 -> R PD Torques/3
  [min_splay_trq] -> Mux7/1  "min_splay_trq"
  [max_splay_trq] -> Mux7/2  "max_splay_trq"
  Gain18/1 -> Gain12/1
  Gain19/1 -> Gain13/1
  Gain20/1 -> Gain10/1
  Gain21/1 -> Gain11/1
  Gain22/1 -> Gain4/1
  Gain23/1 -> Gain7/1
  One-sided PD Ctrl/1 -> [max_splay_trq]
  One-sided PD Ctrl3/1 -> [min_thigh_trq]
  One-sided PD Ctrl1/1 -> [max_thigh_trq]
  One-sided PD Ctrl5/1 -> [min_shin_trq]
  One-sided PD Ctrl4/1 -> [max_shin_trq]

== system atrias_boom_nmStand_fullCtrl/Control/Behavior Control/Virtual Neuromuscular Control/Torque Distribution/mech limit avoidance1/PD Joint Limit/R scale desired torque ==
  note: NOTE: min_splay_angle does not equal delta_phi_min
  phi_thigh [rad] : Inport
  phi_shin [rad] : Inport  Port=2
  Constant : Constant
  Constant1 : Constant  Value=delta_phi_max - delta_phi_max_buffer
  Constant10 : Constant  Value=phi_thigh_max_buffer
  Constant11 : Constant  Value=phi_shin_min_buffer
  Constant12 : Constant  Value=phi_shin_max_buffer
  Constant13 : Constant
  Constant2 : Constant  Value=phi_thigh_max - phi_thigh_max_buffer
  Constant3 : Constant  Value=min_splay_angle
  Constant4 : Constant  Value=phi_thigh_min + phi_thigh_min_buffer
  Constant5 : Constant  Value=phi_shin_max - phi_shin_max_buffer
  Constant6 : Constant  Value=phi_shin_min + phi_shin_min_buffer
  Constant7 : Constant  Value=min_splay_angle - delta_phi_min
  Constant8 : Constant  Value=delta_phi_max_buffer
  Constant9 : Constant  Value=phi_thigh_min_buffer
  Divide{,1..5} (6 alike) : Product  Inputs=/*
  Gain : Gain  Gain=-1
  Gain1 : Gain  Gain=-1
  Gain2 : Gain  Gain=-1
  Mux{,3,7..8} (4 alike) : Mux  Inputs=2
  R scale hip/knee : Scope  NumInputPorts=4
      settings: ShowLegends=on  TimeRange=0.8951752322126555  YMin=0~-1~0~0  YMax=1~1~1~1  SaveName=ScopeData5
  Sum : Sum  Inputs=|+-
  Sum1 : Sum  Inputs=-+|
  Sum2 : Sum  Inputs=+-
  Sum{3..8} (6 alike) : Sum  Inputs=+-|
  [0,1]{,1..5} (6 alike) : Saturate  UpperLimit=1  LowerLimit=0
  max : MinMax  Function=max  Inputs=2
  max1 : MinMax  Function=max  Inputs=4
  scale_hip : Outport
  scale_knee : Outport  Port=2
  wires:
  max/1 -> Sum1/1
  max1/1 -> Sum/2
  [min_shin_scale] -> max1/1
  [max_shin_scale] -> max1/2
  [min_thigh_scale] -> max1/3
  [max_thigh_scale] -> max1/4
  [max_splay_scale] -> max/2
  [min_splay_scale] -> max/1
  Mux3/1 -> R scale hip/knee/4
  Sum1/1 -> scale_knee/1, Mux3/2
  Constant13/1 -> Sum1/2
  Gain2/1 -> Divide5/2
  Constant12/1 -> Divide5/1
  Sum7/1 -> Gain2/1
  "[0,1]5"/1 -> [max_shin_scale]
  Divide5/1 -> "[0,1]5"/1
  Constant11/1 -> Divide4/1
  Sum8/1 -> Divide4/2
  "[0,1]4"/1 -> [min_shin_scale]
  Divide4/1 -> "[0,1]4"/1
  Constant10/1 -> Divide3/1
  Sum5/1 -> Gain1/1
  Gain1/1 -> Divide3/2
  "[0,1]3"/1 -> [max_thigh_scale]
  Divide3/1 -> "[0,1]3"/1
  Constant9/1 -> Divide2/1
  Sum6/1 -> Divide2/2
  "[0,1]2"/1 -> [min_thigh_scale]
  Divide2/1 -> "[0,1]2"/1
  Gain/1 -> Divide1/2
  Constant8/1 -> Divide1/1
  Sum3/1 -> Gain/1
  "[0,1]1"/1 -> [max_splay_scale]
  Divide1/1 -> "[0,1]1"/1
  "[0,1]"/1 -> [min_splay_scale]
  Divide/1 -> "[0,1]"/1
  Sum4/1 -> Divide/2
  Constant7/1 -> Divide/1
  Constant/1 -> Sum/1
  Sum/1 -> scale_hip/1, Mux3/1
  [max_splay_scale] -> Mux7/2  "max_splay_scale"
  [min_splay_scale] -> Mux7/1  "min_splay_scale"
  Mux7/1 -> R scale hip/knee/3
  Mux8/1 -> R scale hip/knee/2
  [max_shin_scale] -> Mux8/2  "max_shin_scale"
  [min_shin_scale] -> Mux8/1  "min_shin_scale"
  Mux/1 -> R scale hip/knee/1
  [max_thigh_scale] -> Mux/2  "max_thigh_scale"
  [min_thigh_scale] -> Mux/1  "min_thigh_scale"
  Constant5/1 -> Sum7/1
  [shin] -> Sum7/2
  Constant6/1 -> Sum8/1
  [shin] -> Sum8/2
  Constant2/1 -> Sum5/1
  [thigh] -> Sum5/2
  Constant4/1 -> Sum6/1
  [thigh] -> Sum6/2
  Constant1/1 -> Sum3/1
  [splay] -> Sum3/2
  Constant3/1 -> Sum4/1
  [splay] -> Sum4/2
  Sum2/1 -> [splay]  "splay angle"
  phi_thigh [rad]/1 -> Sum2/2, [thigh]
  phi_shin [rad]/1 -> Sum2/1, [shin]
